simulink model "Flight_Model_2021a_11_14_2021"  (R2021a)
settings: Solver=VariableStepAuto  StartTime=0.0  StopTime=30  RelTol=1e-3
model workspace (MAT data in the model file):
  bodyLength = 5
  brakesCd = 1
  brakesOn = 1
  dryCG = 3.9
  dryMass = 23
  finArea = 0.2
  finChordAngle = 0.5236
  finSpan = 0.4
  fullBrakesOn = 0
  gravity = 9.8067
  noseLength = 0.5
  propMass = 7.183
  refArea = 0.0182
  rocketCP = 1
  rocketDiam = 0.197
  rocketDiameter = 0.0762
  targetAlt = 3048
  thrust = [0; 2638.366; 2528.97; 3063.078; 2426.009; 2548.275; 2599.755; 2554.71; 2644.801; 2638.366; 2561.145; 2606.19; 2638.366; 2638.366; 2580.45; 2496.795; 2335.919; 2213.653; 2129.998; 1653.805; 888.035; 630.634; 450.453; 289.577; 135.136; 25.74; 0]
  time = [0; 0.045; 0.067; 0.084; 0.124; 0.186; 0.231; 0.298; 0.371; 0.534; 0.979; 1.142; 2.002; 2.289; 2.761; 3.121; 3.436; 3.678; 3.79; 4.004; 4.415; 4.538; 4.656; 4.82; 5.005; 5.219; 5.371]
  totalImpulse = 10831
  vehicleCd = 0.8
  wetCG = 4
  wetMass = 30
undefined symbols (not defined in the file): dryInertia, Earth, wetInertia, WGS84
libraries: aerolibasang x4, aerolibwind2 x3, aerolibbdyn x2, shared6dof x2, aerolibatmos2 x1, aerolibtransform2 x1, aerolibanim x1, sharedschedule x1
settings Model: Creator=alhus  LastModifiedBy=alhus

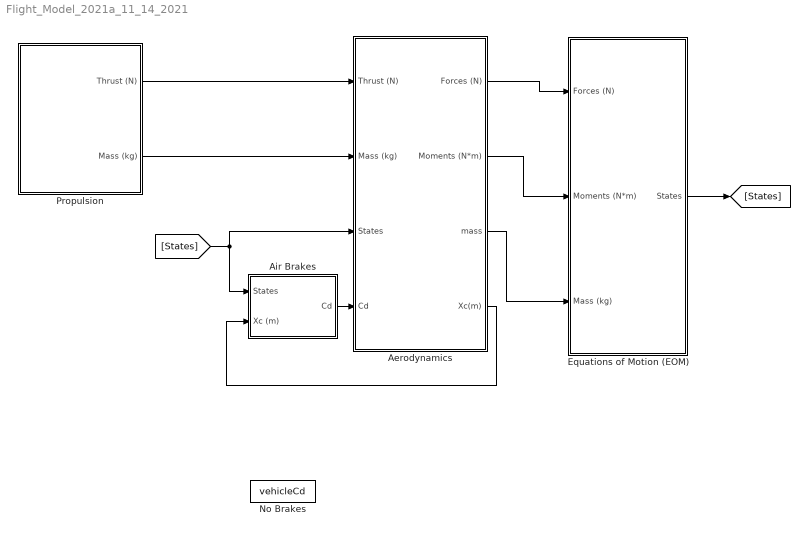
== system Flight_Model_2021a_11_14_2021 ==
  Aerodynamics : Subsystem
  Air Brakes : Subsystem
  Equations of Motion (EOM) : Subsystem
  No Brakes : Constant  Value=vehicleCd
  Propulsion : Subsystem
  wires:
  Propulsion/1(Thrust (N)) -> Aerodynamics/1(Thrust (N))
  Air Brakes/1("Cd ") -> Aerodynamics/4(Cd)
  Propulsion/2(Mass (kg)) -> Aerodynamics/2(Mass (kg))
  [States] -> Air Brakes/1(States), Aerodynamics/3(States)
  Equations of Motion (EOM)/1(States) -> [States]
  Aerodynamics/1(Forces (N)) -> Equations of Motion (EOM)/1(Forces (N))
  Aerodynamics/2(Moments (N*m)) -> Equations of Motion (EOM)/2(Moments (N*m))
  Aerodynamics/3(mass) -> Equations of Motion (EOM)/3(Mass (kg))
  Aerodynamics/4(Xc(m)) -> Air Brakes/2(Xc (m))

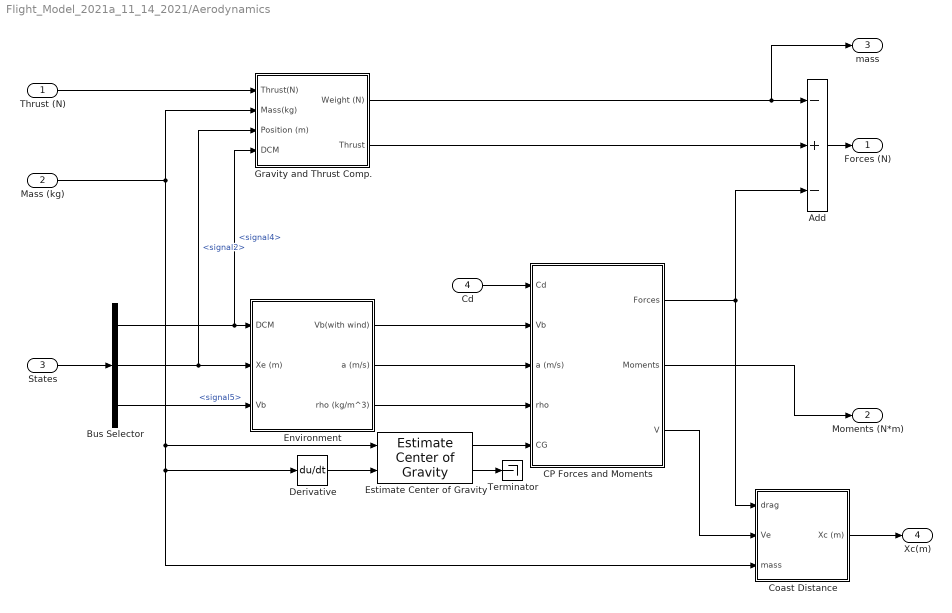
== system Flight_Model_2021a_11_14_2021/Aerodynamics ==
  Thrust (N) : Inport
  Mass (kg) : Inport  Port=2
  States : Inport  Port=3
  Cd : Inport  Port=4
  Add : Sum  Inputs=-+-
  Bus Selector : BusSelector  OutputSignals=signal4,signal2,signal5
  CP Forces and Moments : Subsystem
  Coast Distance : Subsystem
  Derivative : Derivative
  Environment : Subsystem
  Estimate Center of Gravity : aerolibbdyn/Estimate Center of Gravity  fmass=wetMass  emass=dryMass  fcg=[wetCG 0 0]'  ecg=[dryCG 0 0]'
      settings: SourceProductBaseCode=AE
  Gravity and Thrust Comp. : Subsystem
  Terminator : Terminator
  Forces (N) : Outport
  Moments (N*m) : Outport  Port=2
  mass : Outport  Port=3
  Xc(m) : Outport  Port=4
  wires:
  Mass (kg)/1 -> Gravity and Thrust Comp./2(Mass(kg)), Coast Distance/3(mass), Derivative/1, Estimate Center of Gravity/1
  Add/1 -> Forces (N)/1
  States/1 -> Bus Selector/1
  Bus Selector/2 -> Environment/2(Xe (m)), Gravity and Thrust Comp./3(Position (m))  "<signal2>"
  Bus Selector/1 -> Gravity and Thrust Comp./4(DCM), Environment/1(DCM)  "<signal4>"
  Environment/2(a (m/s)) -> CP Forces and Moments/3(a (m/s))
  Environment/3(rho (kg/m^3)) -> CP Forces and Moments/4(rho)
  CP Forces and Moments/2(Moments) -> Moments (N*m)/1
  Cd/1 -> CP Forces and Moments/1(Cd)
  Derivative/1 -> Estimate Center of Gravity/2
  Estimate Center of Gravity/2 -> Terminator/1
  Estimate Center of Gravity/1 -> CP Forces and Moments/5(CG)
  CP Forces and Moments/1(Forces) -> Coast Distance/1(drag), Add/3
  Environment/1(Vb(with wind)) -> CP Forces and Moments/2(Vb)
  Bus Selector/3 -> Environment/3(Vb)  "<signal5>"
  Thrust (N)/1 -> Gravity and Thrust Comp./1(Thrust(N))
  Gravity and Thrust Comp./2(Thrust) -> Add/2
  Gravity and Thrust Comp./1(Weight (N)) -> mass/1, Add/1
  Coast Distance/1(Xc (m)) -> Xc(m)/1
  CP Forces and Moments/3(V) -> Coast Distance/2(Ve)

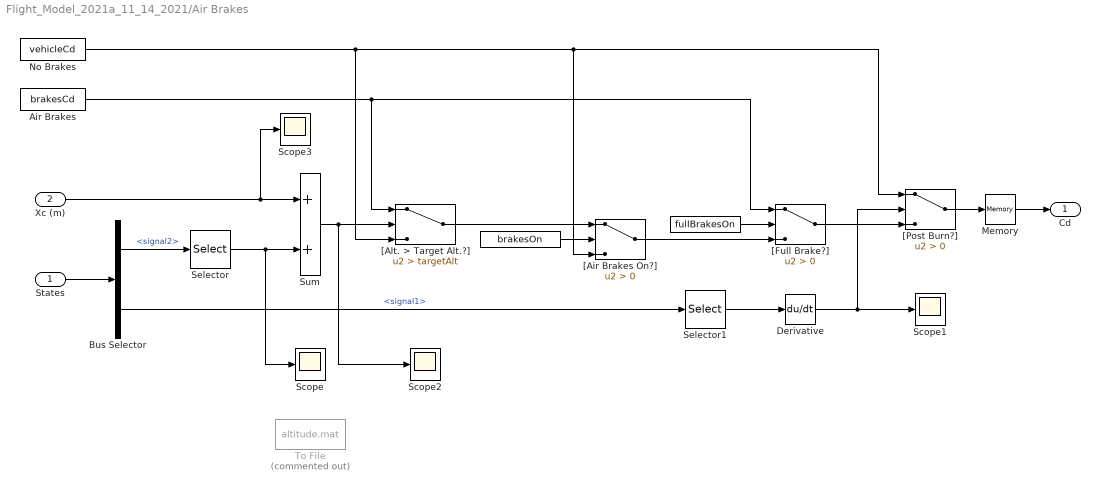
== system Flight_Model_2021a_11_14_2021/Air Brakes ==
  States : Inport
  Xc (m) : Inport  Port=2
  " " : Constant  Value=fullBrakesOn
  "  " : Constant  Value=brakesOn
  Air Brakes : Constant  Value=brakesCd
  Bus Selector : BusSelector  OutputSignals=signal2,signal1
  Derivative : Derivative
  Memory : Memory
  No Brakes : Constant  Value=vehicleCd
  Scope{,1..3} (4 alike) : Scope
  "Selector " : Selector  InputPortWidth=3  IndexOptions=Index vector (dialog)  Indices=1  OutputSizes=1
  Selector1 : Selector  InputPortWidth=3  IndexOptions=Index vector (dialog)  Indices=1  OutputSizes=1
  Sum : Sum
  To File : ToFile  Commented=on  Filename=altitude.mat  SaveFormat=Timeseries
  "[Air Brakes On?]" : Switch  Description=[Air Brakes On?]  Criteria=u2 > Threshold
  "[Alt. > Target Alt.?]" : Switch  Criteria=u2 > Threshold  Threshold=targetAlt
  "[Full Brake?]" : Switch  Criteria=u2 > Threshold
  "[Post Burn?]" : Switch  Criteria=u2 > Threshold
  "Cd " : Outport
  wires:
  Sum/1 -> Scope2/1, "[Alt. > Target Alt.?]"/2
  "[Post Burn?]"/1 -> Memory/1
  No Brakes/1 -> "[Alt. > Target Alt.?]"/3, "[Post Burn?]"/1, "[Air Brakes On?]"/3
  " "/1 -> "[Full Brake?]"/2
  Air Brakes/1 -> "[Alt. > Target Alt.?]"/1, "[Full Brake?]"/1
  "[Full Brake?]"/1 -> "[Post Burn?]"/3
  "Selector "/1 -> Scope/1, Sum/2
  "  "/1 -> "[Air Brakes On?]"/2
  "[Air Brakes On?]"/1 -> "[Full Brake?]"/3
  "[Alt. > Target Alt.?]"/1 -> "[Air Brakes On?]"/1
  States/1 -> Bus Selector/1
  Selector1/1 -> Derivative/1
  Derivative/1 -> "[Post Burn?]"/2, Scope1/1
  Bus Selector/1 -> "Selector "/1  "<signal2>"
  Xc (m)/1 -> Scope3/1, Sum/1
  Bus Selector/2 -> Selector1/1  "<signal1>"
  Memory/1 -> "Cd "/1

== system Flight_Model_2021a_11_14_2021/Equations of Motion (EOM) ==
  Forces (N) : Inport
  Moments (N*m) : Inport  Port=2
  Mass (kg) : Inport  Port=3
  6DOF (Euler Angles) : shared6dof/6DOF (Euler Angles)  units=Metric (MKS)  mtype=Fixed  rep=Euler Angles  xme_0=[0 0 0]  Vm_0=[0 0 0]  eul_0=[0 0 0]  pm_0=[0 0 0]  mass_0=1.0  mass_e=0.5  mass_f=2.0  inertia=eye(3)  inertia_e=eye(3)  inertia_f=2*eye(3)  k_quat=1.0  vre_flag=on  abi_flag=off  aMode=0  xme_statename=''  Vm_statename=''  eul_statename=''  quat_statename=''  pm_statename=''  mass_statename=''
      settings: SourceProductBaseCode=AE,PW,DR,MT,UV,VE
  6DoF Animation : aerolibanim/6DoF Animation  u1=[0 4000 0 2000 0 8000]  u2=.01  u3=100  u4=[4000 0 -5000]  u5=Fly alongside  u6=[2000 500 3150]  u7=10  u8=on
  Bus Creator : BusCreator  Inputs=8
  Custom Variable Mass 6DOF (Euler Angles) : shared6dof/6DOF (Euler Angles)  Commented=on  units=Metric (MKS)  mtype=Custom Variable  rep=Euler Angles  xme_0=[0 0 0]  Vm_0=[0 0 0]  eul_0=[0 0 0]  pm_0=[0 0 0]  mass_0=1.0  mass_e=0.5  mass_f=2.0  inertia=eye(3)  inertia_e=eye(3)  inertia_f=2*eye(3)  k_quat=1.0  vre_flag=off  abi_flag=off  aMode=0  xme_statename=''  Vm_statename=''  eul_statename=''  quat_statename=''  pm_statename=''  mass_statename=''
      settings: SourceProductBaseCode=AE,PW,DR,MT,UV,VE
  Derivative : Derivative  Commented=on
  Estimate Inertia : Subsystem  Commented=on  mask{fmass=wetMass, emass=dryMass, fInertia=[30,0,0;0,wetInertia,0;0,0,wetInertia], eInertia=[30,0,0;0,dryInertia,0;0,0,dryInertia]}
      mask prompts: fmass "Full mass:"; emass "Empty mass:"; fInertia "Full Inertia (3x3)"; eInertia "Empty Inertia (3x3)"
      mask init:
      | inertia(:,:,1)=eInertia;
      | inertia(:,:,2)=fInertia;
  Scope : Scope
  States : Outport
  wires:
  6DOF (Euler Angles)/1 -> Bus Creator/1
  6DOF (Euler Angles)/4 -> Bus Creator/4
  6DOF (Euler Angles)/7 -> Bus Creator/7
  6DOF (Euler Angles)/3 -> 6DoF Animation/2, Bus Creator/3
  6DOF (Euler Angles)/6 -> Bus Creator/6
  6DOF (Euler Angles)/5 -> Bus Creator/5
  Bus Creator/1 -> States/1
  6DOF (Euler Angles)/8 -> Bus Creator/8
  Mass (kg)/1 -> Custom Variable Mass 6DOF (Euler Angles)/3, Derivative/1, Estimate Inertia/1(Mass)
  Derivative/1 -> Estimate Inertia/2(M_dot)
  Estimate Inertia/2(Inertia) -> Custom Variable Mass 6DOF (Euler Angles)/5
  Estimate Inertia/1(Inertia_dot) -> Custom Variable Mass 6DOF (Euler Angles)/4
  6DOF (Euler Angles)/2 -> 6DoF Animation/1, Scope/1, Bus Creator/2
  Forces (N)/1 -> 6DOF (Euler Angles)/1
  Moments (N*m)/1 -> 6DOF (Euler Angles)/2

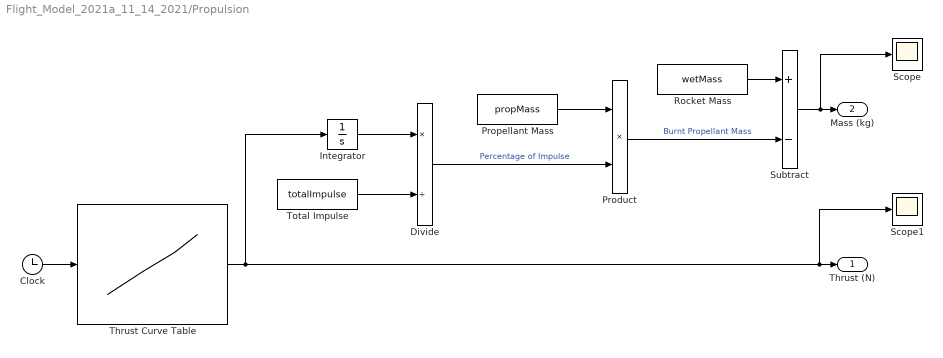
== system Flight_Model_2021a_11_14_2021/Propulsion ==
  Clock : Clock
  Divide : Product  Inputs=*/
  Integrator : Integrator
  Product : Product
  Propellant Mass : Constant  Value=propMass
  Rocket Mass : Constant  Value=wetMass
  Scope : Scope
  Scope1 : Scope
  Subtract : Sum  Inputs=+-
  Thrust Curve Table : Lookup_n-D  NumberOfTableDimensions=1  BreakpointsForDimension1=time  Table=thrust  ExtrapMethod=Clip  InternalRulePriority=Speed  RndMeth=Simplest  InputSameDT=on
  Total Impulse : Constant  Value=totalImpulse
  Thrust (N) : Outport
  Mass (kg) : Outport  Port=2
  wires:
  Total Impulse/1 -> Divide/2
  Integrator/1 -> Divide/1
  Clock/1 -> Thrust Curve Table/1
  Propellant Mass/1 -> Product/1
  Product/1 -> Subtract/2  "Burnt Propellant Mass"
  Rocket Mass/1 -> Subtract/1
  Subtract/1 -> Scope/1, Mass (kg)/1
  Thrust Curve Table/1 -> Scope1/1, Thrust (N)/1, Integrator/1
  Divide/1 -> Product/2  "Percentage of Impulse"

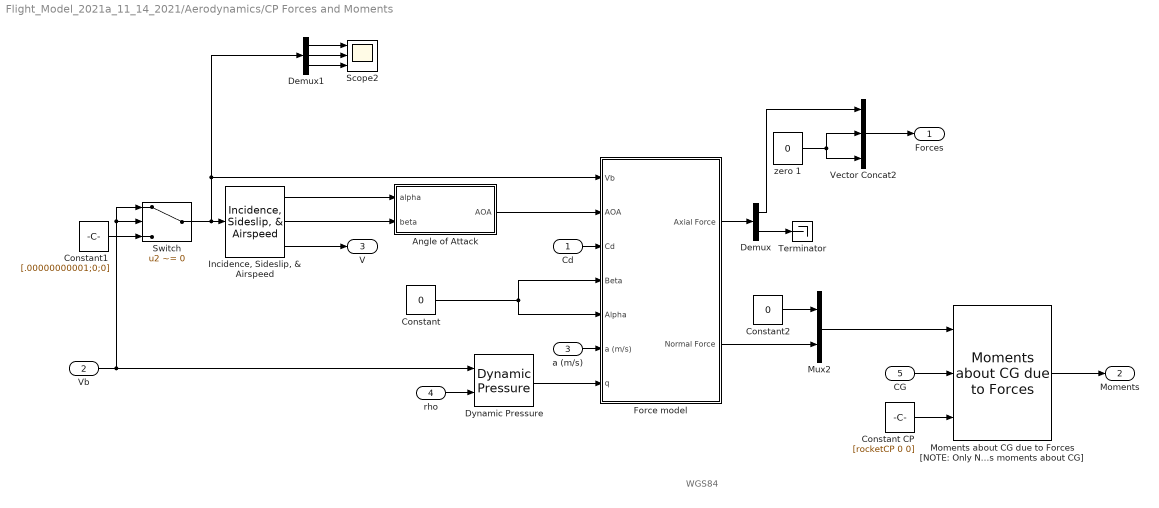
== system Flight_Model_2021a_11_14_2021/Aerodynamics/CP Forces and Moments ==
  note: WGS84
  Cd : Inport
  Vb : Inport  Port=2
  a (m/s) : Inport  Port=3
  rho : Inport  Port=4
  CG : Inport  Port=5
  Angle of Attack : Subsystem
  Constant : Constant  Value=0
  Constant CP : Constant  Value=[rocketCP 0 0]
  Constant1 : Constant  Value=[.00000000001;0;0]  VectorParams1D=off
  Constant2 : Constant  Value=0
  Demux : Demux  Outputs=2
  Demux1 : Demux  Outputs=3
  Dynamic Pressure : aerolibasang/Dynamic Pressure
  Force model : Subsystem
  "Incidence, Sideslip, & Airspeed" : aerolibasang/Incidence, Sideslip, & Airspeed
  Moments about CG due to Forces [NOTE: Only Normal Force applys moments about CG] : aerolibbdyn/Moments about CG  due to Forces
      settings: SourceProductBaseCode=AE
  Mux2 : Mux  Inputs=2
  Scope2 : Scope  NumInputPorts=3
  Switch : Switch  Criteria=u2 ~= 0
  Terminator : Terminator
  Vector Concat2 : Concatenate  NumInputs=3
  zero 1 : Constant  Value=0
  Forces : Outport
  Moments : Outport  Port=2
  V : Outport  Port=3
  wires:
  rho/1 -> Dynamic Pressure/2
  Moments about CG due to Forces [NOTE: Only Normal Force applys moments about CG]/1 -> Moments/1
  Vb/1 -> Dynamic Pressure/1, Switch/1, Switch/2
  "Incidence, Sideslip, & Airspeed"/3 -> V/1
  Constant1/1 -> Switch/3
  Switch/1 -> Demux1/1, Force model/1(Vb), "Incidence, Sideslip, & Airspeed"/1
  Constant CP/1 -> Moments about CG due to Forces [NOTE: Only Normal Force applys moments about CG]/3
  CG/1 -> Moments about CG due to Forces [NOTE: Only Normal Force applys moments about CG]/2
  Force model/1(Axial Force) -> Demux/1
  Dynamic Pressure/1 -> Force model/7("q ")
  a (m/s)/1 -> Force model/6(a (m/s))
  Cd/1 -> Force model/3(Cd)
  Demux/2 -> Terminator/1
  Mux2/1 -> Moments about CG due to Forces [NOTE: Only Normal Force applys moments about CG]/1
  Constant2/1 -> Mux2/1
  Force model/2(Normal Force) -> Mux2/2
  "Incidence, Sideslip, & Airspeed"/2 -> Angle of Attack/2(beta)
  "Incidence, Sideslip, & Airspeed"/1 -> Angle of Attack/1(alpha)
  Angle of Attack/1(AOA) -> Force model/2(AOA)
  Demux1/2 -> Scope2/2
  Demux1/3 -> Scope2/3
  Demux1/1 -> Scope2/1
  Constant/1 -> Force model/4(Beta), Force model/5(Alpha)
  zero 1/1 -> Vector Concat2/3, Vector Concat2/2
  Demux/1 -> Vector Concat2/1
  Vector Concat2/1 -> Forces/1

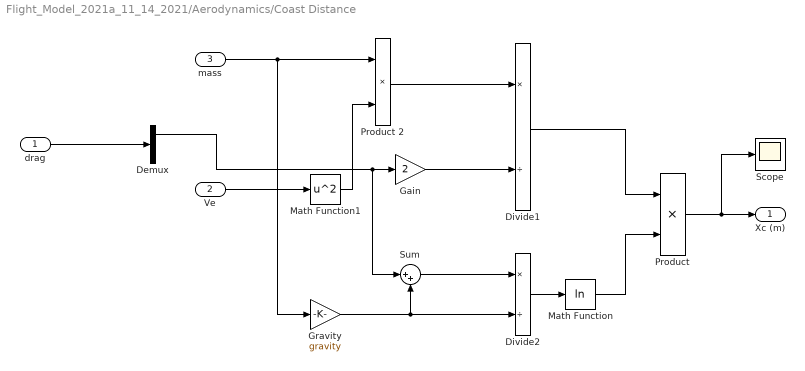
== system Flight_Model_2021a_11_14_2021/Aerodynamics/Coast Distance ==
  drag : Inport
  Ve : Inport  Port=2
  mass : Inport  Port=3
  Demux : Demux  Outputs=3
  Divide1 : Product  Inputs=*/
  Divide2 : Product  Inputs=*/
  Gain : Gain  Gain=2
  Gravity : Gain  Gain=gravity
  Math Function : Math  Operator=log  SignedPower=on  SaturateOnIntegerOverflow=on
  Math Function1 : Math  Operator=square  SignedPower=on  SaturateOnIntegerOverflow=on
  Product : Product
  Product 2 : Product  Inputs=**
  Scope : Scope
  Sum : Sum  Inputs=|++
  Xc (m) : Outport
  wires:
  Math Function/1 -> Product/2
  mass/1 -> Gravity/1, Product 2/1
  Divide1/1 -> Product/1
  Divide2/1 -> Math Function/1
  Product/1 -> Xc (m)/1, Scope/1
  Sum/1 -> Divide2/1
  Gravity/1 -> Sum/2, Divide2/2
  Ve/1 -> Math Function1/1
  Math Function1/1 -> Product 2/2
  Product 2/1 -> Divide1/1
  Gain/1 -> Divide1/2
  drag/1 -> Demux/1
  Demux/1 -> Sum/1, Gain/1

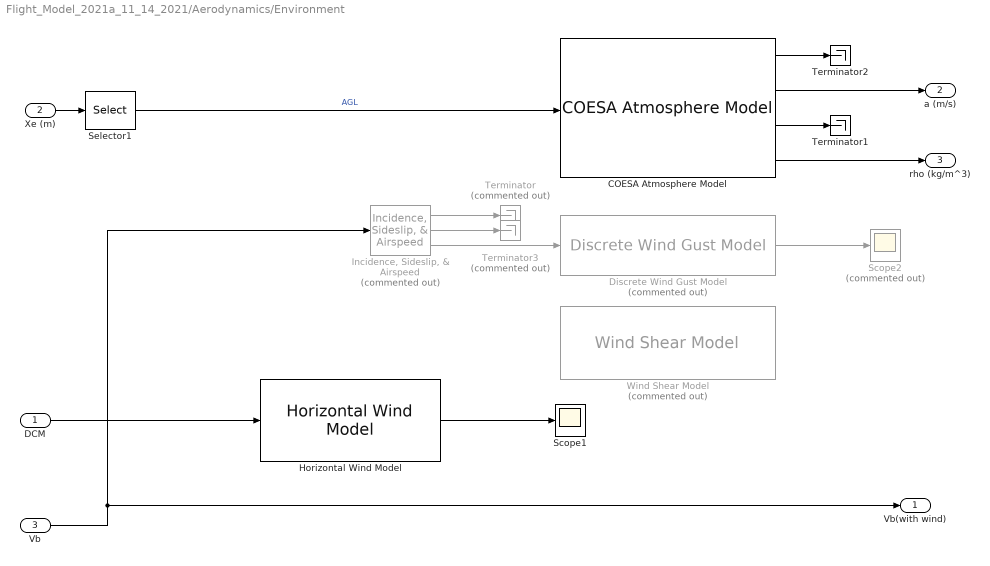
== system Flight_Model_2021a_11_14_2021/Aerodynamics/Environment ==
  DCM : Inport
  Xe (m) : Inport  Port=2
  Vb : Inport  Port=3
  COESA Atmosphere Model : aerolibatmos2/COESA Atmosphere Model  units=Metric (MKS)  spec=1976 COESA-extended U.S. Standard Atmosphere  model=Profile  profile_var=High temperature  profile_percent=1%  profile_alt=5 km (16404 ft)  envelope_var=High temperature  envelope_percent=1%  action=Warning
  Discrete Wind Gust Model : aerolibwind2/Discrete Wind Gust Model  Commented=on  units=Metric (MKS)  Gx=on  Gy=on  Gz=on  t_0=2  d_m=[120 120 80]  v_m=[3.5 3.5 3]
  Horizontal Wind Model : aerolibwind2/Horizontal Wind Model  units=Metric (MKS)  Vw_source=Internal  Vwind=1  W_source=Internal  Wdeg=90
      settings: SourceProductBaseCode=AE
  "Incidence, Sideslip, & Airspeed" : aerolibasang/Incidence, Sideslip, & Airspeed  Commented=on
  Scope1 : Scope
  Scope2 : Scope  Commented=on
  Selector1 : Selector  InputPortWidth=3  IndexOptions=Index vector (dialog)  Indices=1  OutputSizes=1
  Terminator : Terminator  Commented=on
  Terminator1 : Terminator
  Terminator2 : Terminator
  Terminator3 : Terminator  Commented=on
  Wind Shear Model : aerolibwind2/Wind Shear Model  Commented=on  units=Metric (MKS)  phase=Category C - Terminal Flight Phase  W_20=15  Wdeg=0
  Vb(with wind) : Outport
  a (m/s) : Outport  Port=2
  rho (kg/m^3) : Outport  Port=3
  wires:
  "Incidence, Sideslip, & Airspeed"/3 -> Discrete Wind Gust Model/1
  "Incidence, Sideslip, & Airspeed"/1 -> Terminator/1
  Xe (m)/1 -> Selector1/1
  DCM/1 -> Horizontal Wind Model/1
  Selector1/1 -> COESA Atmosphere Model/1  "AGL"
  COESA Atmosphere Model/2 -> a (m/s)/1
  COESA Atmosphere Model/4 -> rho (kg/m^3)/1
  COESA Atmosphere Model/1 -> Terminator2/1
  COESA Atmosphere Model/3 -> Terminator1/1
  Horizontal Wind Model/1 -> Scope1/1
  "Incidence, Sideslip, & Airspeed"/2 -> Terminator3/1
  Discrete Wind Gust Model/1 -> Scope2/1
  Vb/1 -> Vb(with wind)/1, "Incidence, Sideslip, & Airspeed"/1

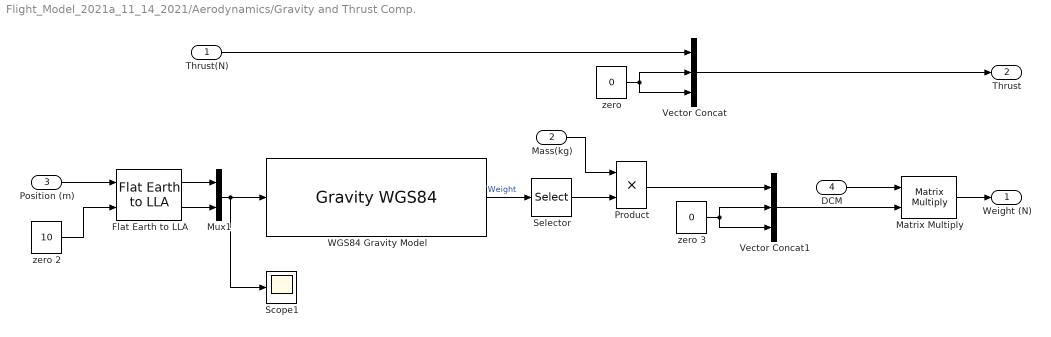
== system Flight_Model_2021a_11_14_2021/Aerodynamics/Gravity and Thrust Comp. ==
  Thrust(N) : Inport
  Mass(kg) : Inport  Port=2
  Position (m) : Inport  Port=3
  DCM : Inport  Port=4
  Flat Earth to LLA : aerolibtransform2/Flat Earth to LLA  units=Metric (MKS)  ptype=Earth (WGS84)  F=1/298.257223563  R=6378137  refPosPort=off  LL0=[0 10]  psi=0
  Matrix Multiply : Product  Multiplication=Matrix(*)
  Mux1 : Mux  Inputs=2
  Product : Product
  Scope1 : Scope
  Selector : Selector  InputPortWidth=3  IndexOptions=Index vector (dialog)  Indices=[3]  OutputSizes=1
  Vector Concat : Concatenate  NumInputs=3
  Vector Concat1 : Concatenate  NumInputs=3
  "WGS84 Gravity Model  " : GravityWGS84
  "zero " : Constant  Value=0
  zero 2 : Constant  Value=10
  zero 3 : Constant  Value=0
  Weight (N) : Outport
  Thrust : Outport  Port=2
  wires:
  "zero "/1 -> Vector Concat/3, Vector Concat/2
  Thrust(N)/1 -> Vector Concat/1
  DCM/1 -> Matrix Multiply/1
  Matrix Multiply/1 -> Weight (N)/1
  Vector Concat/1 -> Thrust/1
  Mass(kg)/1 -> Product/1
  Mux1/1 -> Scope1/1, "WGS84 Gravity Model  "/1
  Flat Earth to LLA/1 -> Mux1/1
  Flat Earth to LLA/2 -> Mux1/2
  Position (m)/1 -> Flat Earth to LLA/1
  zero 2/1 -> Flat Earth to LLA/2
  zero 3/1 -> Vector Concat1/3, Vector Concat1/2
  Product/1 -> Vector Concat1/1
  Vector Concat1/1 -> Matrix Multiply/2
  Selector/1 -> Product/2
  "WGS84 Gravity Model  "/1 -> Selector/1  "Weight"

== system Flight_Model_2021a_11_14_2021/Equations of Motion (EOM)/Estimate Inertia ==
  Mass : Inport
  M_dot : Inport  Port=2
  Constant : Constant  Value=emass
  Constant1 : Constant  Value=fmass
  Interpolate Inertia : sharedschedule/Interpolate Matrix(x)   matrix=inertia  aMode=aMode
      settings: SourceProductBaseCode=AE,PW,DR,MT,UV,VE
  Mux : Mux  Inputs=2
  PreLook-Up Index Search1 : PreLookup  BreakpointsDataSource=Input port  BreakpointsData=[emass fmass]  BeginIndexSearchUsingPreviousIndexResult=on  IndexDataTypeStr=int32  FractionDataTypeStr=double
      settings: InputPortMap=u0,p1
  Product : Product  SaturateOnIntegerOverflow=on  OutDataTypeStr=Inherit: Same as first input
  slope : Constant  Value=(fInertia - eInertia)/(fmass - emass)
  Inertia_dot : Outport
  Inertia : Outport  Port=2
  wires:
  M_dot/1 -> Product/2
  slope/1 -> Product/1
  Product/1 -> Inertia_dot/1
  Constant1/1 -> Mux/2
  Constant/1 -> Mux/1
  Mux/1 -> PreLook-Up Index Search1/2
  PreLook-Up Index Search1/2 -> Interpolate Inertia/2
  PreLook-Up Index Search1/1 -> Interpolate Inertia/1
  Interpolate Inertia/1 -> Inertia/1
  Mass/1 -> PreLook-Up Index Search1/1

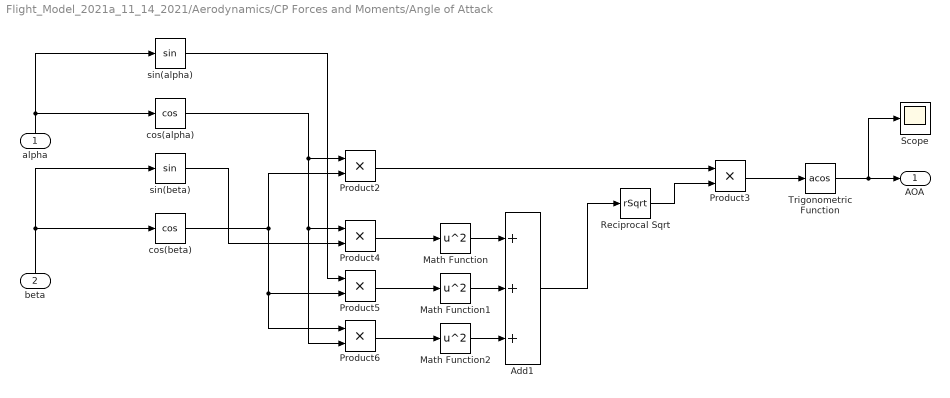
== system Flight_Model_2021a_11_14_2021/Aerodynamics/CP Forces and Moments/Angle of Attack ==
  alpha : Inport
  beta : Inport  Port=2
  Add1 : Sum  Inputs=+++
  Math Function : Math  Operator=square  SignedPower=on  SaturateOnIntegerOverflow=on
  Math Function1 : Math  Operator=square  SignedPower=on  SaturateOnIntegerOverflow=on
  Math Function2 : Math  Operator=square  SignedPower=on  SaturateOnIntegerOverflow=on
  Product{2..6} (5 alike) : Product
  Reciprocal Sqrt : Sqrt  Operator=rSqrt  SaturateOnIntegerOverflow=on
  Scope : Scope
  Trigonometric Function : Trigonometry  Operator=acos
  cos(alpha) : Trigonometry  Operator=cos
  cos(beta) : Trigonometry  Operator=cos
  sin(alpha) : Trigonometry
  sin(beta) : Trigonometry
  AOA : Outport
  wires:
  Product3/1 -> Trigonometric Function/1
  Math Function2/1 -> Add1/3
  Product5/1 -> Math Function1/1
  Product6/1 -> Math Function2/1
  alpha/1 -> sin(alpha)/1, cos(alpha)/1
  cos(alpha)/1 -> Product6/2, Product4/1, Product2/1
  beta/1 -> cos(beta)/1, sin(beta)/1
  cos(beta)/1 -> Product6/1, Product5/2, Product2/2
  Reciprocal Sqrt/1 -> Product3/2
  Math Function/1 -> Add1/1
  Math Function1/1 -> Add1/2
  sin(beta)/1 -> Product4/2
  Add1/1 -> Reciprocal Sqrt/1
  sin(alpha)/1 -> Product5/1
  Product2/1 -> Product3/1
  Product4/1 -> Math Function/1
  Trigonometric Function/1 -> Scope/1, AOA/1

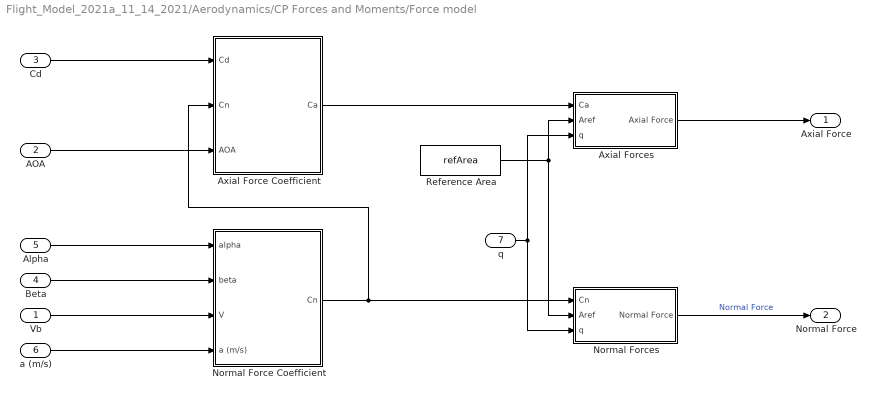
== system Flight_Model_2021a_11_14_2021/Aerodynamics/CP Forces and Moments/Force model ==
  Vb : Inport
  AOA : Inport  Port=2
  Cd : Inport  Port=3
  Beta : Inport  Port=4
  Alpha : Inport  Port=5
  a (m/s) : Inport  Port=6
  "q " : Inport  Port=7
  Axial Force Coefficient : Subsystem
  Axial Forces : Subsystem
  Normal Force Coefficient : Subsystem
  Normal Forces : Subsystem
  Reference Area : Constant  Value=refArea
  Axial Force : Outport
  Normal Force : Outport  Port=2
  wires:
  Reference Area/1 -> Normal Forces/2(Aref), Axial Forces/2(Aref)
  Axial Force Coefficient/1(Ca) -> Axial Forces/1(Ca)
  Normal Force Coefficient/1(Cn) -> Normal Forces/1(Cn), Axial Force Coefficient/2(Cn)
  Axial Forces/1(Axial Force) -> Axial Force/1
  Normal Forces/1(Normal Force) -> Normal Force/1  "Normal Force"
  Cd/1 -> Axial Force Coefficient/1(Cd)
  AOA/1 -> Axial Force Coefficient/3(AOA)
  Beta/1 -> Normal Force Coefficient/2(beta)
  Alpha/1 -> Normal Force Coefficient/1(alpha)
  a (m/s)/1 -> Normal Force Coefficient/4(a (m/s))
  Vb/1 -> Normal Force Coefficient/3(V)
  "q "/1 -> Axial Forces/3("q "), Normal Forces/3("q ")

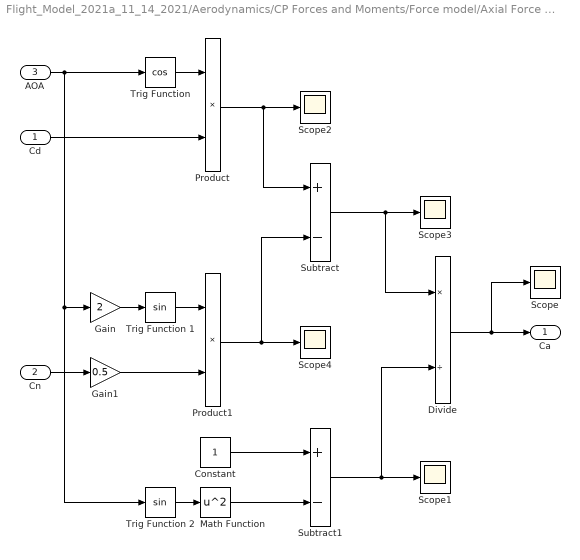
== system Flight_Model_2021a_11_14_2021/Aerodynamics/CP Forces and Moments/Force model/Axial Force Coefficient ==
  Cd : Inport
  Cn : Inport  Port=2
  AOA : Inport  Port=3
  Constant : Constant
  Divide : Product  Inputs=*/
  Gain : Gain  Gain=2
  Gain1 : Gain  Gain=0.5
  Math Function : Math  Operator=square  SignedPower=on  SaturateOnIntegerOverflow=on
  Product : Product
  Product1 : Product
  Scope{,1..4} (5 alike) : Scope
  Subtract : Sum  Inputs=+-
  Subtract1 : Sum  Inputs=+-
  Trig Function : Trigonometry  Operator=cos
  Trig Function 1 : Trigonometry
  Trig Function 2 : Trigonometry
  Ca : Outport
  wires:
  AOA/1 -> Trig Function/1, Trig Function 2/1, Gain/1
  Cd/1 -> Product/2
  Trig Function/1 -> Product/1
  Gain/1 -> Trig Function 1/1
  Trig Function 1/1 -> Product1/1
  Gain1/1 -> Product1/2
  Cn/1 -> Gain1/1
  Product1/1 -> Scope4/1, Subtract/2
  Divide/1 -> Scope/1, Ca/1
  Trig Function 2/1 -> Math Function/1
  Math Function/1 -> Subtract1/2
  Constant/1 -> Subtract1/1
  Subtract/1 -> Scope3/1, Divide/1
  Subtract1/1 -> Scope1/1, Divide/2
  Product/1 -> Scope2/1, Subtract/1

== system Flight_Model_2021a_11_14_2021/Aerodynamics/CP Forces and Moments/Force model/Axial Forces ==
  Ca : Inport
  Aref : Inport  Port=2
  "q " : Inport  Port=3
  Product : Product  Inputs=3
  Scope : Scope
  Axial Force : Outport
  wires:
  Ca/1 -> Product/1
  Aref/1 -> Product/2
  Product/1 -> Axial Force/1, Scope/1
  "q "/1 -> Product/3

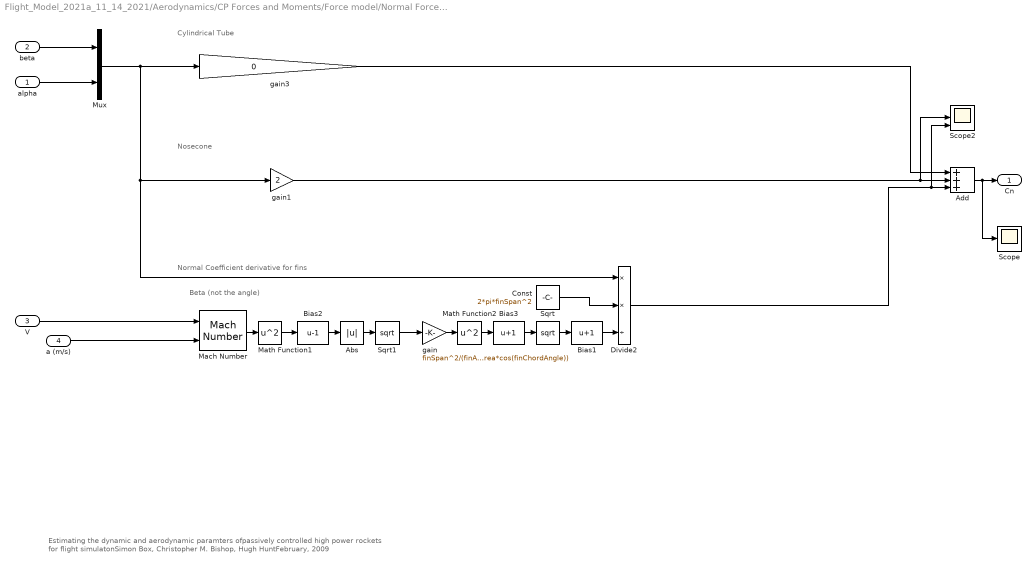
== system Flight_Model_2021a_11_14_2021/Aerodynamics/CP Forces and Moments/Force model/Normal Force Coefficient ==
  note: Estimating the dynamic and aerodynamic paramters ofpassively controlled high power rockets for flight simulatonSimon Box, Christopher M. Bishop, Hugh HuntFebruary, 2009
  note: Cylindrical Tube
  note: Normal Coefficient derivative for fins
  note: Beta (not the angle)
  note: Nosecone
  alpha : Inport
  beta : Inport  Port=2
  V : Inport  Port=3
  a (m/s) : Inport  Port=4
  Abs : Abs
  Add : Sum  Inputs=+++
  Bias1 : Bias  Bias=1
  Bias2 : Bias  Bias=-1
  Bias3 : Bias  Bias=1
  Const : Constant  Value=2*pi*finSpan^2
  Divide2 : Product  Inputs=**/
  Mach Number : aerolibasang/Mach Number
      settings: SourceProductBaseCode=AE
  Math Function1 : Math  Operator=square  SignedPower=on  SaturateOnIntegerOverflow=on
  Math Function2 : Math  Operator=square  SignedPower=on  SaturateOnIntegerOverflow=on
  Mux : Mux  Inputs=2
  Scope : Scope
  Scope2 : Scope  NumInputPorts=3
  Sqrt : Sqrt  SaturateOnIntegerOverflow=on
  Sqrt1 : Sqrt  SaturateOnIntegerOverflow=on
  gain : Gain  Gain=finSpan^2/(finArea*cos(finChordAngle))
  gain1 : Gain  Gain=2
  gain3 : Gain  Gain=0
  Cn : Outport
  wires:
  Sqrt1/1 -> gain/1
  Math Function2/1 -> Bias3/1
  Sqrt/1 -> Bias1/1
  Bias3/1 -> Sqrt/1
  gain/1 -> Math Function2/1
  a (m/s)/1 -> Mach Number/2
  Bias1/1 -> Divide2/3
  Add/1 -> Scope/1, Cn/1
  V/1 -> Mach Number/1
  Mach Number/1 -> Math Function1/1
  Math Function1/1 -> Bias2/1
  Bias2/1 -> Abs/1
  Abs/1 -> Sqrt1/1
  Const/1 -> Divide2/2
  gain1/1 -> Scope2/2, Add/2
  gain3/1 -> Add/1
  Divide2/1 -> Add/3, Scope2/3
  beta/1 -> Mux/1
  alpha/1 -> Mux/2
  Mux/1 -> gain3/1, Divide2/1, gain1/1

== system Flight_Model_2021a_11_14_2021/Aerodynamics/CP Forces and Moments/Force model/Normal Forces ==
  Cn : Inport
  Aref : Inport  Port=2
  "q " : Inport  Port=3
  Product : Product  Inputs=3
  Scope : Scope
  Normal Force : Outport
  wires:
  Cn/1 -> Product/1
  Aref/1 -> Product/2
  Product/1 -> Normal Force/1, Scope/1
  "q "/1 -> Product/3
